simulink library "fuselage_cl"  (R2018b)
settings: Solver=VariableStepAuto  StartTime=0.0  StopTime=10.0  RelTol=1e-3
libraries: vrlib x2, dynamicPressure_ul x1, localApparentWind_ul x1
settings Model: Creator=mcobb  LastModifiedBy=jldanie5

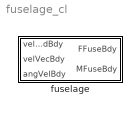
== system fuselage_cl ==
  fuselage : Subsystem  mask{len=0, diam=0, sideCD=0, endCD=0}
      mask prompts: len "Length"; diam "Diameter"; sideCD "Sideways drag coeff"; endCD "End-ways drag coeff"

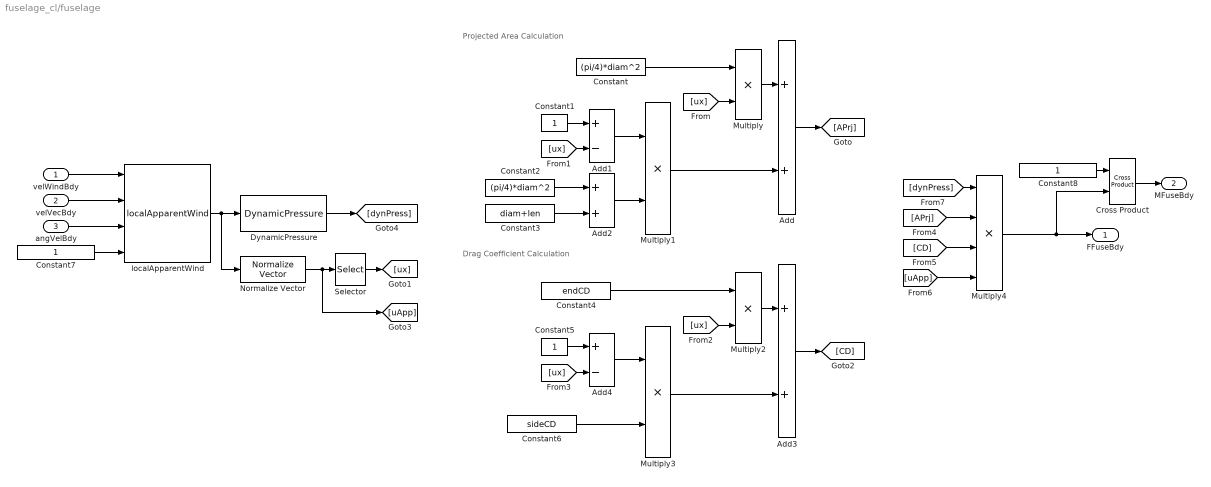
== system fuselage_cl/fuselage ==
  note: Drag Coefficient Calculation
  note: Projected Area Calculation
  velWindBdy : Inport
  velVecBdy : Inport  Port=2
  angVelBdy : Inport  Port=3
  Add : Sum
  Add1 : Sum  Inputs=+-
  Add2 : Sum
  Add3 : Sum
  Add4 : Sum  Inputs=+-
  Constant : Constant  Value=(pi/4)*diam^2
  Constant{1,5,7..8} (4 alike) : Constant
  Constant2 : Constant  Value=(pi/4)*diam^2
  Constant3 : Constant  Value=diam+len
  Constant4 : Constant  Value=endCD
  Constant6 : Constant  Value=sideCD
  Cross Product : vrlib/Utilities/Cross Product
      settings: SourceProductBaseCode=VR
  DynamicPressure : dynamicPressure_ul/DynamicPressure  rho=fluidDensity
  Multiply{,1..3} (4 alike) : Product
  Multiply4 : Product  Inputs=4
  Normalize Vector : vrlib/Utilities/Normalize Vector  maxzero=0
      settings: SourceProductName=Simulink 3D Animation  SourceProductBaseCode=VR
  Selector : Selector  InputPortWidth=3  IndexOptions=Index vector (dialog)  Indices=1  OutputSizes=1
  localApparentWind : localApparentWind_ul/localApparentWind  SystemSampleTime=-1
  FFuseBdy : Outport
  MFuseBdy : Outport  Port=2
  wires:
  Normalize Vector/1 -> [uApp], Selector/1
  Add/1 -> [APrj]
  Selector/1 -> [ux]
  Multiply1/1 -> Add/2
  Multiply/1 -> Add/1
  Constant/1 -> Multiply/1
  [ux] -> Multiply/2
  Add1/1 -> Multiply1/1
  Constant1/1 -> Add1/1
  [ux] -> Add1/2
  Add2/1 -> Multiply1/2
  Constant2/1 -> Add2/1
  Constant3/1 -> Add2/2
  [ux] -> Add4/2
  Constant5/1 -> Add4/1
  Add4/1 -> Multiply3/1
  [ux] -> Multiply2/2
  Multiply2/1 -> Add3/1
  Multiply3/1 -> Add3/2
  Constant6/1 -> Multiply3/2
  Constant4/1 -> Multiply2/1
  Add3/1 -> [CD]
  Multiply4/1 -> Cross Product/2, FFuseBdy/1
  [dynPress] -> Multiply4/1
  [APrj] -> Multiply4/2
  [CD] -> Multiply4/3
  [uApp] -> Multiply4/4
  angVelBdy/1 -> localApparentWind/3
  localApparentWind/1 -> Normalize Vector/1, DynamicPressure/1
  velVecBdy/1 -> localApparentWind/2
  Constant7/1 -> localApparentWind/4
  velWindBdy/1 -> localApparentWind/1
  DynamicPressure/1 -> [dynPress]
  Constant8/1 -> Cross Product/1
  Cross Product/1 -> MFuseBdy/1
